simulink model "boucle (1)"  (R2014a)
settings: Solver=ode45  StartTime=0.0  StopTime=0.003  FixedStep=Delta  MaxStep=1e-6  RelTol=1e-3
undefined symbols (not defined in the file): a, b, K, Kd, tau, Te
settings Model: Creator=aymeric  LastModifiedBy=aymeric

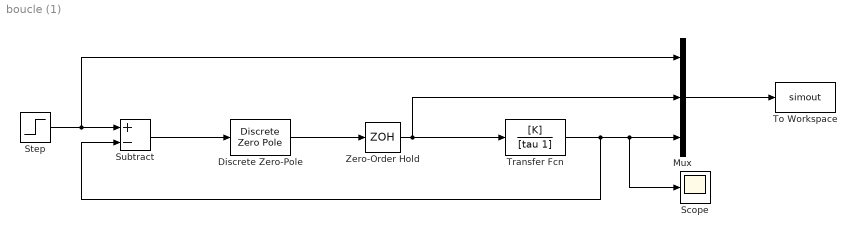
== system boucle (1) ==
  Discrete Zero-Pole : DiscreteZeroPole  Zeros=[0 a]  Poles=[1 -b]  Gain=Kd  SampleTime=Te
  Mux : Mux  Inputs=3
  Scope : Scope
  Step : Step  Time=0  SampleTime=Te
  Subtract : Sum  Inputs=+-  SampleTime=Te
  To Workspace : ToWorkspace  VariableName=simout  SaveFormat=Timeseries  SampleTime=-1
  Transfer Fcn : TransferFcn  Numerator=[K]  Denominator=[tau 1]
  Zero-Order Hold : ZeroOrderHold  SampleTime=Te
  wires:
  Step/1 -> Mux/1, Subtract/1
  Subtract/1 -> Discrete Zero-Pole/1
  Discrete Zero-Pole/1 -> Zero-Order Hold/1
  Transfer Fcn/1 -> Subtract/2, Scope/1, Mux/3
  Mux/1 -> To Workspace/1
  Zero-Order Hold/1 -> Transfer Fcn/1, Mux/2
